simulink model "meu_esboco"  (R2017a)
settings: Solver=VariableStepAuto  StartTime=0.0  StopTime=inf  RelTol=1e-3
settings Model: Creator=dscat  LastModifiedBy=dscat

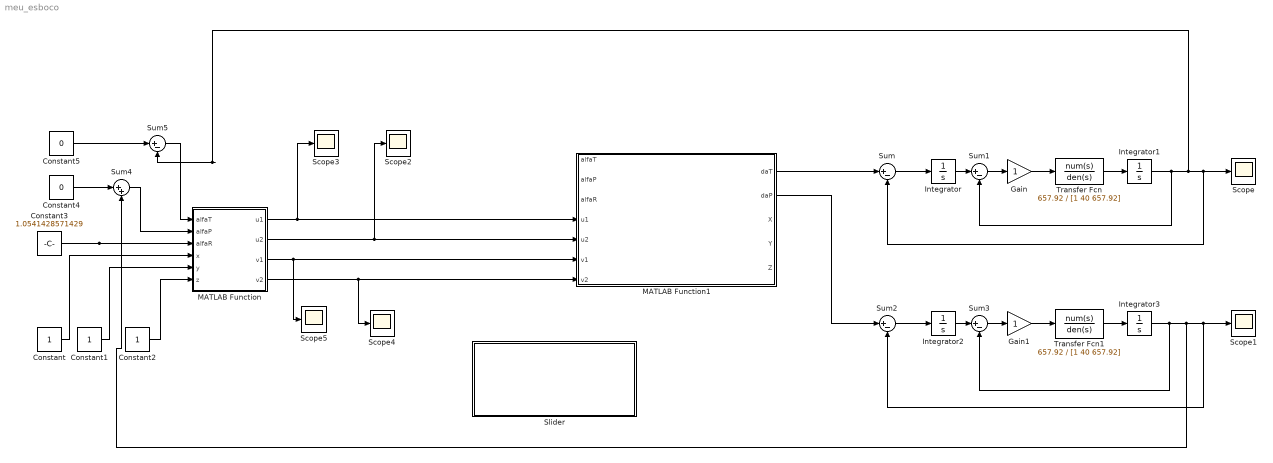
== system meu_esboco ==
  Constant : Constant
  Constant1 : Constant
  Constant2 : Constant
  Constant3 : Constant  Value=1.0541428571429
  Constant4 : Constant  Value=0
  Constant5 : Constant  Value=0
  Gain : Gain
  Gain1 : Gain
  Integrator{,1..3} (4 alike) : Integrator
  MATLAB Function : MATLAB Function  TreatAsAtomicUnit=on
  MATLAB Function1 : MATLAB Function  TreatAsAtomicUnit=on
  Scope{,1..5} (6 alike) : Scope
  Slider : Subsystem  DialogController=hmiCreateDDGDialog  IsWebBlock=on  mask(MWDashboardBlock){webBlockId=0ac94893-dbea-46a7-ad2a-ffe1e3efa20e, webBlockType=slider, ShowInLibBrowser=on, ShowInitialText=on, HMISrcModelName=meu_esboco}
      mask prompts: webBlockId "WebBlock Id"; webBlockType "WebBlock Type"; HMISrcModelName "Source Model"
      mask help: SimulinkHMI:dialogs:SliderDialogDesc
      mask Help: helpview([docroot '/mapfiles/simulink.map'], 'hmi_slider')
      mask Display:
      | if strcmp(get_param(bdroot(gcb),'BlockDiagramType'), 'library')
      |     image([(matlabroot) '/toolbox/simulink/hmi/icons/Slider.png']);
      | end
  Sum{,1..3,5} (5 alike) : Sum  Inputs=|+-
  Sum4 : Sum  Inputs=|++
  Transfer Fcn : TransferFcn  Numerator=657.92  Denominator=[1 40 657.92]
  Transfer Fcn1 : TransferFcn  Numerator=657.92  Denominator=[1 40 657.92]
  wires:
  MATLAB Function/1(u1) -> Scope3/1, MATLAB Function1/4(u1)
  MATLAB Function/2(u2) -> Scope2/1, MATLAB Function1/5(u2)
  MATLAB Function/3(v1) -> MATLAB Function1/6(v1), Scope5/1
  MATLAB Function/4(v2) -> Scope4/1, MATLAB Function1/7(v2)
  MATLAB Function1/1(daT) -> Sum/1
  Sum/1 -> Integrator/1
  Integrator/1 -> Sum1/1
  Sum1/1 -> Gain/1
  Gain/1 -> Transfer Fcn/1
  Transfer Fcn/1 -> Integrator1/1
  Gain1/1 -> Transfer Fcn1/1
  MATLAB Function1/2(daP) -> Sum2/1
  Transfer Fcn1/1 -> Integrator3/1
  Sum3/1 -> Gain1/1
  Integrator3/1 -> Sum4/2, Sum2/2, Scope1/1, Sum3/2
  Integrator2/1 -> Sum3/1
  Sum2/1 -> Integrator2/1
  Sum5/1 -> MATLAB Function/1(alfaT)
  Sum4/1 -> MATLAB Function/2(alfaP)
  Constant3/1 -> MATLAB Function/3(alfaR)
  Constant/1 -> MATLAB Function/4(x)
  Constant1/1 -> MATLAB Function/5(y)
  Constant2/1 -> MATLAB Function/6(z)
  Constant4/1 -> Sum4/1
  Constant5/1 -> Sum5/1
  Integrator1/1 -> Sum5/2, Sum/2, Scope/1, Sum1/2

== system meu_esboco/Slider ==

== matlab function meu_esboco/MATLAB Function1 ==
  data: alfaT input; daT output; alfaP input; alfaR input; u1 input; u2 input; v1 input; v2 input; daP output; X output; Y output; Z output
function [daT, daP, X,Y,Z  ] = image2real( alfaT,alfaP,alfaR, u1,u2,v1,v2)
% daT -> Delta Alfa Tilt
% daP -> Delta Alfa Pan
% AlfaR -> Lido dos encoders


l = 0.15; %Tamanho do alvo (m) 
f = 664;

X = (l*(f*cos(alfaP-alfaR) - u2*sin(alfaP-alfaR))*(- cos(alfaP-alfaR)*sin(alfaP-alfaR)*f^2 + (u1 - cos(alfaP-alfaR)^2*(u1 + u2))*f + u1*u2*cos(alfaP-alfaR)*sin(alfaP-alfaR)))/(f*(u2*cos(alfaP-alfaR) + f*sin(alfaP-alfaR))*(u1 - u2));

%  X = (l*(f*cos(alfaT) - v2*sin(alfaT))*(- cos(alfaT)*sin(alfaT)*f^2 + (v1 - cos(alfaT)^2*(v1 + v2))*f + v1*v2*cos(alfaT)*sin(alfaT)))/(f*(f*sin(alfaT) + v2*cos(alfaT))*(v1 - v2));

Y = -(l*(2*cos(alfaP-alfaR)*sin(alfaP-alfaR)*f^2 + (u1 + u2)*(2*cos(alfaP-alfaR)^2 - 1)*f - 2*u1*u2*cos(alfaP-alfaR)*sin(alfaP-alfaR)))/(2*f*(u1 - u2));

Z  = -(l*(2*cos(alfaT)*sin(alfaT)*f^2 + (v1 + v2)*(2*cos(alfaT)^2 - 1)*f - 2*v1*v2*cos(alfaT)*sin(alfaT)))/(2*f*(v1 - v2));
 
daP = double(atan(Y/X)-alfaR);
daT = double(atan(Z/(sqrt((X)^2+(Y)^2))));


end

== matlab function meu_esboco/MATLAB Function ==
  data: alfaT input; u1 output; alfaP input; alfaR input; x input; y input; z input; u2 output; v1 output; v2 output
function [u1, u2, v1, v2] = real2image(alfaT,alfaP,alfaR,x,y,z)
L = 0.15;
f = 664;
u1 = f*(-sin(alfaP-alfaR)*(-x)+cos(alfaP-alfaR)*((L/2)-y))/((cos(alfaP-alfaR)*(-x)+sin(alfaP-alfaR)*((L/2)-y)));
u2 = f*(-sin(alfaP-alfaR)*(-x)+cos(alfaP-alfaR)*((-L/2)-y))/((cos(alfaP-alfaR)*(-x)+sin(alfaP-alfaR)*((-L/2)-y)));
v1 = f*(-sin(alfaT)*(-x)+cos(alfaT)*((L/2)-z))/((cos(alfaT)*(-x)+sin(alfaT)*((L/2)-z)));
v2 = f*(-sin(alfaT)*(-x)+cos(alfaT)*((-L/2)-z))/((cos(alfaT)*(-x)+sin(alfaT)*((-L/2)-z)));

end
